simulink model "MotorPC"  (R2020b)
settings: Solver=VariableStepAuto  StartTime=0.0  StopTime=10.0  RelTol=1e-3
values from neighbouring files (symbols this model uses):
  b = 3.5077E-6    (= 3.5077e-06)    [Init.m]    (also in Prob4_MotorPC.sldd = 3.5077E-6)
  J = 3.2284E-6    (= 3.2284e-06)    [Init.m]    (also in Prob4_MotorPC.sldd = 3.2284E-6)
  K = 0.0274    [Init.m]    (also in Prob4_MotorPC.sldd)
  L = 2.75E-6    (= 2.75e-06)    [Init.m]    (also in Prob4_MotorPC.sldd = 2.75E-6)
  R = 4    [Init.m]    (also in Prob4_MotorPC.sldd = 4.0)
settings Model: Creator=Rasika Shejul  LastModifiedBy=Rasika Shejul

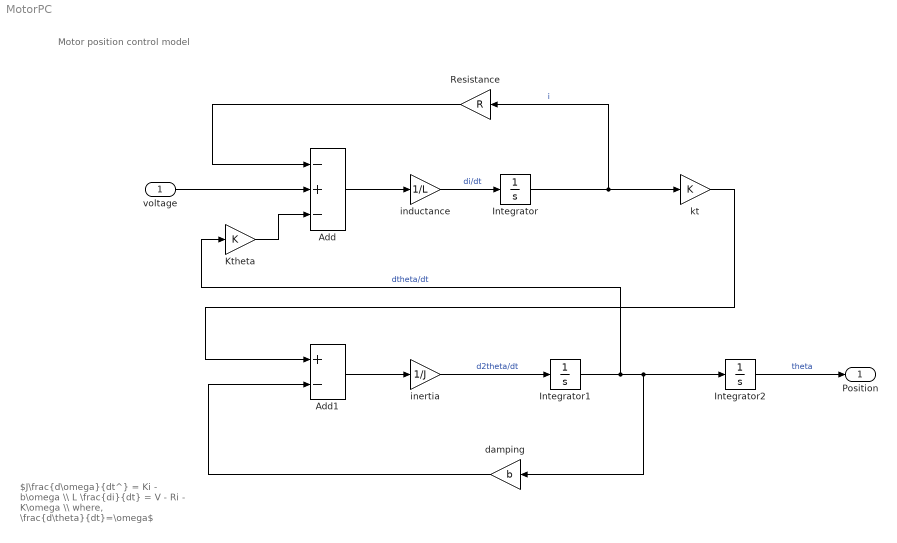
== system MotorPC ==
  note: $J\frac{d\omega}{dt^} = Ki - b\omega \\ L \frac{di}{dt} = V - Ri - K\omega \\ where, \frac{d\theta}{dt}=\omega$
  note: Motor position control model
  voltage : Inport
  Add : Sum  Inputs=-+-
  Add1 : Sum  Inputs=+-
  Integrator : Integrator
  Integrator1 : Integrator
  Integrator2 : Integrator
  Ktheta : Gain  Gain=K
  Resistance : Gain  Gain=R
  damping : Gain  Gain=b
  inductance : Gain  Gain=1/L
  inertia : Gain  Gain=1/J
  kt : Gain  Gain=K
  Position : Outport
  wires:
  Add1/1 -> inertia/1
  inertia/1 -> Integrator1/1  "d2theta/dt"
  inductance/1 -> Integrator/1  "di/dt"
  Integrator1/1 -> Ktheta/1, damping/1, Integrator2/1  "dtheta/dt"
  Add/1 -> inductance/1
  Integrator/1 -> Resistance/1, kt/1  "i"
  Integrator2/1 -> Position/1  "theta"
  kt/1 -> Add1/1
  damping/1 -> Add1/2
  Resistance/1 -> Add/1
  Ktheta/1 -> Add/3
  voltage/1 -> Add/2
